simulink model "tilp_pil_fxp"  (R2013b)
settings: Solver=FixedStepDiscrete  StartTime=0.0  StopTime=10  RelTol=1e-3
settings Model: Creator=bas  LastModifiedBy=peselnikmg
settings DataIOCC: SaveOutput=off  SaveTime=off
settings OptimizationCC: InlineParams=on  ExpressionDepthLimit=2147483647  OptimizeModelRefInitCode=on  LifeSpan=Inf
settings DebuggingCC: FcnCallInpInsideContextMsg=EnableAllAsWarning  StateNameClashWarn=warning
settings HardwareCC: ProdBitPerInt=16  ProdBitPerPointer=16  ProdIntDivRoundTo=Zero  ProdEndianess=LittleEndian  ProdWordSize=16  ProdHWDeviceType=Texas Instruments->MSP430
settings RTWCC: SystemTargetFile=launchpad.tlc  TemplateMakefile=launchpad_tmf  Description=TI LaunchPad  GenerateReport=on  ProcessScript=launchpad_make_rtw_hook  IncludeHyperlinkInReport=on  CodeProfilingSaveOptions=AllData  GenerateTraceInfo=on  GenerateTraceReport=on  GenerateTraceReportSl=on  GenerateTraceReportSf=on  GenerateTraceReportEml=on
settings CodeAppCC: IgnoreCustomStorageClasses=off  CustomSymbolStrType=$N$R$M  InternalIdentifier=Classic
settings STFCustomTargetCC: CombineOutputUpdateFcns=on  ERTCustomFileBanners=on  SupportNonFinite=off  PurelyIntegerCode=on  SupportContinuousTime=off  SupportNonInlinedSFcns=off  MATLABClassNameForMDSCustomization=Simulink.SoftwareTarget.ERTCustomization  GRTInterface=off  SystemTargetFile=launchpad.tlc
settings ERTTargetCC: CodeReplacementLibrary=ANSI_C  ParMdlRefBuildCompliant=off  CompOptLevelCompliant=off  ConcurrentExecutionCompliant=off  ERTFirstTimeCompliant=off  SupportNonFinite=off  PurelyIntegerCode=on  ModelStepFunctionPrototypeControlCompliant=off  CPPClassGenCompliant=off  ExtModeMexFile=noextcomm  InlinedParameterPlacement=NonHierarchical  ERTCustomFileTemplate=launchpad_srmain.tlc

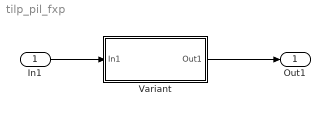
== system tilp_pil_fxp ==
  In1 : Inport  OutMin=-2*pi  OutMax=2*pi  OutDataTypeStr=fixdt(1,16,12)  PortDimensions=1
  Variant : Subsystem  Variant=on
  Out1 : Outport
  wires:
  In1/1 -> Variant/1(In1)
  Variant/1(Out1) -> Out1/1

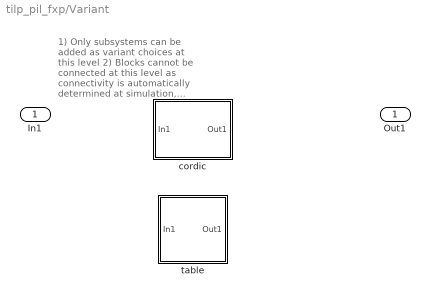
== system tilp_pil_fxp/Variant ==
  note: 1) Only subsystems can be added as variant choices at this level
      | 2) Blocks cannot be connected at this level as connectivity is
      | automatically determined at simulation, based on the active variant
  In1 : Inport
  cordic : Subsystem  VariantControl=cordic == 1
  table : Subsystem  VariantControl=cordic == 0
  Out1 : Outport

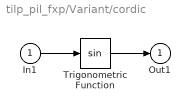
== system tilp_pil_fxp/Variant/cordic ==
  In1 : Inport
  Trigonometric Function : Trigonometry  ApproximationMethod=CORDIC  NumberOfIterations=8
  Out1 : Outport
  wires:
  In1/1 -> Trigonometric Function/1
  Trigonometric Function/1 -> Out1/1

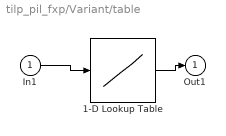
== system tilp_pil_fxp/Variant/table ==
  In1 : Inport
  1-D Lookup Table : Lookup_n-D  NumberOfTableDimensions=1  BreakpointsForDimension1=[-6.283203125;-6.033203125;-5.783203125;-5.533203125;-5.283203125;-5.033203125;-4.783203125;-4.533203125;-4.283203125;-4.033203125;-3.783203125;-3.533203125;-3.283203125;-3.033203125;-2.783203125;-2.533203125;-2.283203125;-2.033203125;-1.783203125;-1.533203125;-1.283203125;-1.033203125;-0.783203125;-0.533203125;-0.283203125;-0.033203125;0.216796875;0.466796875;0.716796875;0.966796875;1.216796875;1.466796875;1.716796875;1.966796875;2.216796875;2.466796875;2.716796875;2.966796875;3.216796875;3.466796875;3.716796875;3.966796875;4.216796875;4.466796875;4.716796875;4.966796875;5.216796875;5.466796875;5.716796875;5.966796875;6.216796875;6.466796875]  IndexSearchMethod=Evenly spaced points  Table=[-1.78178204125803e-05;0.247386695307725;0.479409901919615;0.681625722814269;0.841461357664869;0.948979000847722;0.997493726062959;0.98398912267395;0.909304841510941;0.77808438944921;0.598486418642023;0.381677461045537;0.14113764754598;-0.108177421288899;-0.350766542016859;-0.571546698072349;-0.756790848683145;-0.894981409779732;-0.977526361588228;-0.99929345880516;-0.9589293287528;-0.858943617537316;-0.705552952409166;-0.508294421990405;-0.279432606296305;-0.0331970245525354;0.215102587390736;0.450028162282502;0.656973165719524;0.823070759709924;0.937993800340001;0.994596929564079;0.989360838959806;0.922611083280363;0.798497839036709;0.624737866623186;0.412134719531717;0.17390703172184;-0.0751333530154805;-0.31950230976478;-0.544006160377195;-0.734686342788375;-0.879687286800447;-0.969993536015401;-0.99999028524826;-0.967812481918619;-0.875460785986858;-0.728677178607843;-0.536587953553552;-0.311136288468819;-0.0663396759312193;0.182581616344785]  ExtrapMethod=Clip  RemoveProtectionInput=on  InternalRulePriority=Speed  OutDataTypeStr=fixdt(1,16,14)  RndMeth=Simplest  InputSameDT=on
  Out1 : Outport
  wires:
  In1/1 -> 1-D Lookup Table/1
  1-D Lookup Table/1 -> Out1/1
